simulink model "ukol7"  (R2017b)
settings: Solver=VariableStepAuto  StartTime=0.0  StopTime=10.0  RelTol=1e-3
settings Model: Creator=ladislav  LastModifiedBy=ladislav

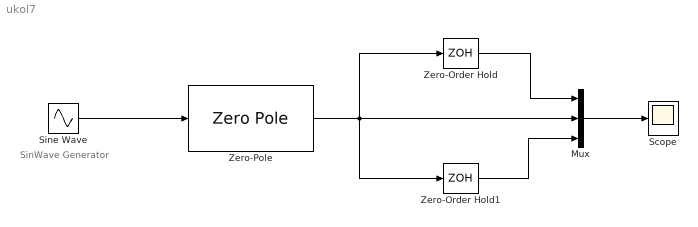
== system ukol7 ==
  note: SinWave Generator
  Mux : Mux  Inputs=3
  "Scope " : Scope
  Sine Wave : Sin  Amplitude=3  Frequency=2*pi  Samples=2*pi
  "Zero-Order Hold " : ZeroOrderHold  SampleTime=0.1
  "Zero-Order Hold1 " : ZeroOrderHold  SampleTime=0.5
  "Zero-Pole " : ZeroPole  Zeros=[3]  Poles=[-1 -7]
  wires:
  Sine Wave/1 -> "Zero-Pole "/1
  Mux/1 -> "Scope "/1
  "Zero-Pole "/1 -> "Zero-Order Hold1 "/1, "Zero-Order Hold "/1, Mux/2
  "Zero-Order Hold "/1 -> Mux/1
  "Zero-Order Hold1 "/1 -> Mux/3
